simulink model "qbot_platform_alpha_driver_physical"  (R2024a)
settings: Solver=ode1  StartTime=0.0  StopTime=inf  FixedStep=1/480  RelTol=1e-3  EnableMultiTasking=on
undefined symbols (not defined in the file): HIL, qc_get_step_size
libraries: quarc_library x26, simulink x14
settings Model: SimulationMode=external  ExtModeTrigDuration=10000  Creator=mbohra  LastModifiedBy=mbohra
settings SolverCC: AlgebraicLoopSolver=TrustRegion  PositivePriorityOrder=on
settings DataIOCC: ReturnWorkspaceOutputs=off
settings OptimizationCC: ReuseModelBlockBuffer=off
settings DebuggingCC: UnconnectedInputMsg=warning  UnconnectedOutputMsg=warning  UnconnectedLineMsg=warning  ArithmeticOperatorsInVariantConditions=warning
settings HardwareCC: ProdBitPerLong=64  ProdLargestAtomicInteger=LongLong  ProdLargestAtomicFloat=Double  ProdLongLongMode=on  ProdHWDeviceType=ARM Compatible->ARM 64-bit (LP64)
settings ModelReferenceCC: EnableRefExpFcnMdlSchedulingChecks=on
settings SFSimCC: SimUseLocalCustomCode=off  CustomCodeUndefinedFunction=UseInterfaceOnly
settings RTWCC: Description=QUARC Linux Raspberry Pi Arm64 Target (QBot Platform Alpha) Using Toolchain  SystemTargetFile=quarc_linux_pi_arm64.tlc  TemplateMakefile=quarc_default_tmf  RTWUseLocalCustomCode=off  Toolchain=QUARC linux_pi_arm64 | gmake (64-bit Windows)  BuildConfiguration=Faster Runs  GPUComputeCapability=3.5
settings CodeAppCC: StateflowObjectComments=on
settings STFCustomTargetCC: ConcurrentExecutionCompliant=on  SystemTargetFile=quarc_linux_pi_arm64.tlc
settings GRTTargetCC: ParMdlRefBuildCompliant=off  CompOptLevelCompliant=off  CombineOutputUpdateFcns=off  MatFileLogging=off  CPPClassGenCompliant=off  GRTInterface=on  ExtMode=on  ExtModeMexFile=quarc_comm  ExtModeMexArgs='-w -d /tmp -uri %u', 'tcpip://192.168.3.29:17099'
settings ConfigComp: CovMetricSettings=dswe

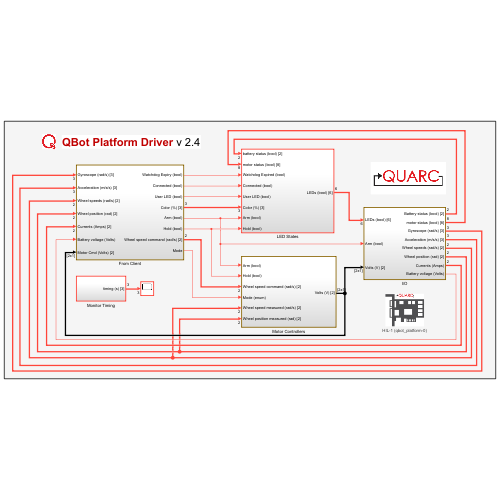
[thumbnail: Simulink's stored preview of the top-level diagram]
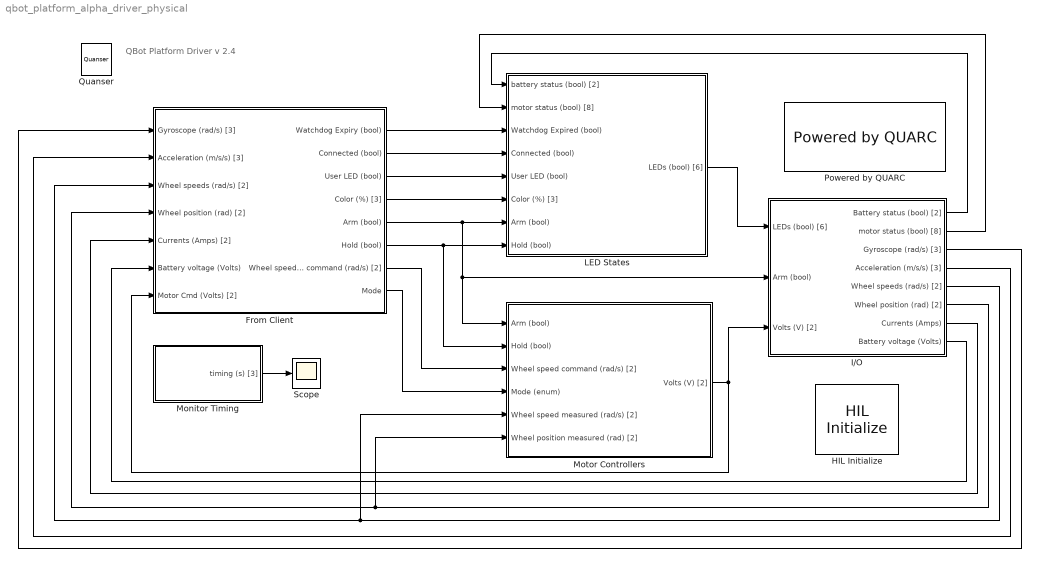
== system qbot_platform_alpha_driver_physical ==
  note: QBot Platform Driver v 2.4
  From Client : Subsystem
  HIL Initialize : quarc_library/Data Acquisition/Generic/Configuration/HIL Initialize  object_name=HIL-1  board_type=qbot_platform  board_number=0  board_options=usb_update_rate=0.002  exclusive=off  active=on  hardware_clocks=[]  clock_modes=[]  initial_clock_frequencies=[]  set_clock_params_at_start=off  set_clock_params_at_switch_in=off  set_clock_frequencies_at_start=off  set_clock_frequencies_at_switch_in=off  analog_input_channels=[0:5]  analog_input_configurations=[]  analog_input_maximums=[18.0 18.0 16.5 16.5 16.5 18.0]  analog_input_minimums=[0 0 0 0 0 0]  set_analog_input_params_at_start=off  set_analog_input_params_at_switch_in=off  analog_output_channels=[]  analog_output_maximums=[]  analog_output_minimums=[]  initial_analog_outputs=[]  final_analog_outputs=[]  watchdog_analog_outputs=[]  set_analog_output_params_at_start=off  set_analog_output_params_at_switch_in=off  set_analog_outputs_at_start=off  set_analog_outputs_at_switch_in=off  set_analog_outputs_at_terminate=off  set_analog_outputs_at_switch_out=off  set_analog_outputs_on_watchdog=off  digital_input_channels=[28:40]  digital_output_channels=[28:30]  digital_output_configuration=[]  initial_digital_outputs=[1]  final_digital_outputs=[0]  watchdog_digital_outputs=[0]  set_digital_output_params_at_start=off  set_digital_output_params_at_switch_in=off  set_digital_outputs_at_start=on  set_digital_outputs_at_switch_in=off  set_digital_outputs_at_terminate=on  set_digital_outputs_at_switch_out=off  set_digital_outputs_on_watchdog=on  encoder_channels=[0:1]  quadrature=[4]  encoder_filter_frequency=[]  initial_encoder_counts=[0]  set_encoder_params_at_start=on  set_encoder_params_at_switch_in=off  set_encoder_counts_at_start=on  set_encoder_counts_at_switch_in=off  pwm_channels=[0:1]  pwm_modes=0  pwm_frequency=[4095 4095]  pwm_configuration=[0]  pwm_alignment=[0]  pwm_polarity=[1]  pwm_leading_deadband=[]  pwm_trailing_deadband=[]  initial_pwm_outputs=[0]  final_pwm_outputs=[0]  watchdog_pwm_outputs=[0]  set_pwm_params_at_start=on  set_pwm_params_at_switch_in=off  set_pwm_outputs_at_start=on  set_pwm_outputs_at_switch_in=off  set_pwm_outputs_at_terminate=on  set_pwm_outputs_at_switch_out=off  set_pwm_outputs_on_watchdog=on  other_output_channels=[11000:11005]  initial_other_outputs=[0 1 0 0 1 0]  final_other_outputs=[1 0 0 1 0 0]  watchdog_other_outputs=[0 0 1 0 0 1]  set_other_outputs_at_start=on  set_other_outputs_at_switch_in=off  set_other_outputs_at_terminate=on  set_other_outputs_at_switch_out=off  set_other_outputs_on_watchdog=on
  I/O : Subsystem
  LED States : Subsystem
  Monitor Timing : Subsystem
  Motor Controllers : Subsystem
  Powered by QUARC : quarc_library/Logos/Powered by QUARC
  Quanser : quarc_library/Logos/Quanser
  Scope : Scope
  wires:
  Monitor Timing/1(timing (s) [3]) -> Scope/1
  From Client/8(Mode) -> Motor Controllers/4(Mode (enum))
  I/O/3(Gyroscope (rad/s) [3]) -> From Client/1(Gyroscope (rad/s) [3])
  I/O/4(Acceleration (m/s/s) [3]) -> From Client/2(Acceleration (m/s/s) [3])
  From Client/5(Arm (bool)) -> Motor Controllers/1(Arm (bool)), I/O/2(Arm (bool)), LED States/7(Arm (bool))
  From Client/3(User LED (bool)) -> LED States/5(User LED (bool))
  From Client/2(Connected (bool)) -> LED States/4(Connected (bool))
  From Client/1(Watchdog Expiry (bool)) -> LED States/3(Watchdog Expired (bool))
  From Client/4(Color (%) [3]) -> LED States/6(Color (%) [3])
  From Client/6(Hold (bool)) -> Motor Controllers/2(Hold (bool)), LED States/8(Hold (bool))
  LED States/1(LEDs (bool) [6]) -> I/O/1(LEDs (bool) [6])
  I/O/5(Wheel speeds (rad/s) [2]) -> Motor Controllers/5(Wheel speed measured (rad/s) [2]), From Client/3(Wheel speeds (rad/s) [2])
  I/O/6(Wheel position (rad) [2]) -> Motor Controllers/6(Wheel position measured (rad) [2]), From Client/4(Wheel position (rad) [2])
  Motor Controllers/1(Volts (V) [2]) -> I/O/3(Volts (V) [2]), From Client/7(Motor Cmd (Volts) [2])
  From Client/7(Wheel speed command (rad/s) [2]) -> Motor Controllers/3(Wheel speed command (rad/s) [2])
  I/O/1(Battery status (bool) [2]) -> LED States/1(battery status (bool) [2])
  I/O/2(motor status (bool) [8]) -> LED States/2(motor status (bool) [8])
  I/O/7(Currents (Amps)) -> From Client/5(Currents (Amps) [2])
  I/O/8(Battery voltage (Volts)) -> From Client/6(Battery voltage (Volts))

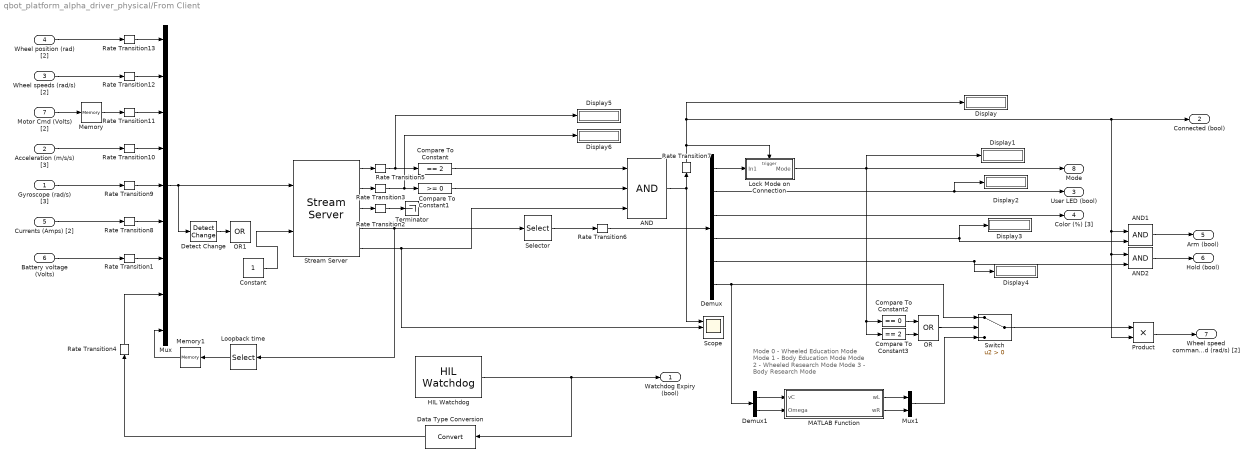
== system qbot_platform_alpha_driver_physical/From Client ==
  note: Mode 0 - Wheeled Education Mode
      | Mode 1 - Body Education Mode
      | Mode 2 - Wheeled Research Mode
      | Mode 3 - Body Research Mode
  Gyroscope (rad/s) [3] : Inport
  Acceleration (m/s/s) [3] : Inport  Port=2
  Wheel speeds (rad/s) [2] : Inport  Port=3
  Wheel position (rad) [2] : Inport  Port=4
  Currents (Amps) [2] : Inport  Port=5
  Battery voltage (Volts) : Inport  Port=6
  Motor Cmd (Volts) [2] : Inport  Port=7
  AND : Logic  Inputs=3  IconShape=distinctive  AllPortsSameDT=off  OutDataTypeStr=boolean
  AND1 : Logic  IconShape=distinctive  AllPortsSameDT=off  OutDataTypeStr=boolean
  AND2 : Logic  IconShape=distinctive  AllPortsSameDT=off  OutDataTypeStr=boolean
  Compare To Constant : simulink/Logic and Bit Operations/Compare To Constant  relop===  const=2  OutDataTypeStr=boolean
  Compare To Constant1 : simulink/Logic and Bit Operations/Compare To Constant  relop=>=  const=0  OutDataTypeStr=boolean
  Compare To Constant2 : simulink/Logic and Bit Operations/Compare To Constant  relop===  const=0  OutDataTypeStr=boolean
  Compare To Constant3 : simulink/Logic and Bit Operations/Compare To Constant  relop===  const=2  OutDataTypeStr=boolean
  Constant : Constant
  Data Type Conversion : DataTypeConversion  SaturateOnIntegerOverflow=off  RndMeth=Floor
  Demux : Demux  Outputs=[1 1 3 1 1 2]
  Demux1 : Demux  Outputs=2
  Detect Change : simulink/Logic and Bit Operations/Detect Change  vinit=0  OutDataTypeStr=boolean
  Display{,1..6} (7 alike) : Display
  HIL Watchdog : quarc_library/Data Acquisition/Generic/Watchdog/HIL Watchdog  object_name=HIL-1  timeout=0.1  sample_time=qc_get_step_size  active=off
      settings: AttributesFormatString=(%<object_name>)  SourceProductName=QUARC Targets
  Lock Mode on Connection : Subsystem  TreatAsAtomicUnit=on
  Loopback time : Selector  InputPortWidth=10  IndexOptions=Index vector (dialog)  Indices=10  OutputSizes=1
  MATLAB Function : MATLAB Function  TreatAsAtomicUnit=on
  Memory : Memory
  Memory1 : Memory  InheritSampleTime=on
  Mux : Mux  Inputs=9
  Mux1 : Mux  Inputs=2
  OR : Logic  Operator=OR  IconShape=distinctive  AllPortsSameDT=off  OutDataTypeStr=boolean
  OR1 : Logic  Operator=OR  Inputs=1  IconShape=distinctive  AllPortsSameDT=off
  Product : Product
  Rate Transition{1..13} (13 alike) : RateTransition
  Scope : Scope  NumInputPorts=3
  Selector : Selector  InputPortWidth=10  IndexOptions=Index vector (dialog)  Indices=1:9  OutputSizes=1
  Stream Server : quarc_library/Communications/Basic/Stream Server  uri_source=Specify via dialog (do not evaluate)  uri=tcpip://localhost:18888?nagle='off'  send_buffer_size=1460  receive_buffer_size=1460  byte_order=little endian (Intel - LSB first)  optimization=Minimum latency  send_options=Send most recent data  receive_options=Receive most recent data  default_value=zeros(10,1)  sample_time=qc_get_step_size*8  active=off  implementation=Use blocking I/O in a separate thread  send_fifo_size=1000  receive_fifo_size=1000  send_priority=0  receive_priority=0  send_dimensions=off  receive_dimensions=off  max_dimensions=-1  data_type=Inherited via back propagation  type_expr=BusObject
      settings: AttributesFormatString="\"tcpip://localhost:18888?nagle='off'\""
  Switch : Switch  Criteria=u2 > Threshold  SaturateOnIntegerOverflow=off  InputSameDT=off
  Terminator : Terminator
  Watchdog Expiry (bool) : Outport
  Connected (bool) : Outport  Port=2
  User LED (bool) : Outport  Port=3
  Color (%) [3] : Outport  Port=4
  Arm (bool) : Outport  Port=5
  Hold (bool) : Outport  Port=6
  Wheel speed command (rad/s) [2] : Outport  Port=7
  Mode : Outport  Port=8
  wires:
  HIL Watchdog/1 -> Data Type Conversion/1, Watchdog Expiry (bool)/1
  Demux/3 -> Color (%) [3]/1
  Demux/5 -> AND2/2, Display4/1
  Demux/2 -> Display2/1, User LED (bool)/1
  Demux/6 -> Demux1/1, Switch/1
  Stream Server/2 -> Rate Transition3/1
  Stream Server/1 -> Rate Transition5/1
  Compare To Constant1/1 -> AND/2
  Compare To Constant/1 -> AND/1
  Gyroscope (rad/s) [3]/1 -> Rate Transition9/1
  Acceleration (m/s/s) [3]/1 -> Rate Transition10/1
  Wheel position (rad) [2]/1 -> Rate Transition13/1
  Motor Cmd (Volts) [2]/1 -> Memory/1
  Detect Change/1 -> OR1/1
  Stream Server/3 -> Rate Transition2/1
  Lock Mode on Connection/1(Mode) -> Mode/1, Display1/1, Compare To Constant3/1, Compare To Constant2/1
  Data Type Conversion/1 -> Rate Transition4/1
  Memory/1 -> Rate Transition11/1
  Compare To Constant2/1 -> OR/1
  Compare To Constant3/1 -> OR/2
  OR/1 -> Switch/2
  Mux1/1 -> Switch/3
  Demux/1 -> Lock Mode on Connection/1(In1)
  MATLAB Function/1(wL) -> Mux1/1
  MATLAB Function/2(wR) -> Mux1/2
  Selector/1 -> Rate Transition6/1
  Loopback time/1 -> Memory1/1
  Memory1/1 -> Mux/9
  Switch/1 -> Product/1
  Wheel speeds (rad/s) [2]/1 -> Rate Transition12/1
  Demux/4 -> AND1/2, Display3/1
  AND/1 -> Scope/1, Rate Transition7/1
  Demux1/1 -> MATLAB Function/1(vC)
  Demux1/2 -> MATLAB Function/2(Omega)
  AND2/1 -> Hold (bool)/1
  Currents (Amps) [2]/1 -> Rate Transition8/1
  Battery voltage (Volts)/1 -> Rate Transition1/1
  Product/1 -> Wheel speed command (rad/s) [2]/1
  AND1/1 -> Arm (bool)/1
  Stream Server/5 -> AND/3, Scope/2
  Stream Server/4 -> Selector/1, Loopback time/1
  Rate Transition2/1 -> Terminator/1
  Rate Transition3/1 -> Display6/1, Compare To Constant1/1
  Rate Transition5/1 -> Display5/1, Compare To Constant/1
  Constant/1 -> Stream Server/2
  Mux/1 -> Stream Server/1, Detect Change/1
  Rate Transition1/1 -> Mux/7
  Rate Transition8/1 -> Mux/6
  Rate Transition9/1 -> Mux/5
  Rate Transition10/1 -> Mux/4
  Rate Transition11/1 -> Mux/3
  Rate Transition12/1 -> Mux/2
  Rate Transition13/1 -> Mux/1
  Rate Transition6/1 -> Demux/1
  Rate Transition7/1 -> Lock Mode on Connection/Trigger, Product/2, AND2/1, AND1/1, Connected (bool)/1, Display/1
  Rate Transition4/1 -> Mux/8

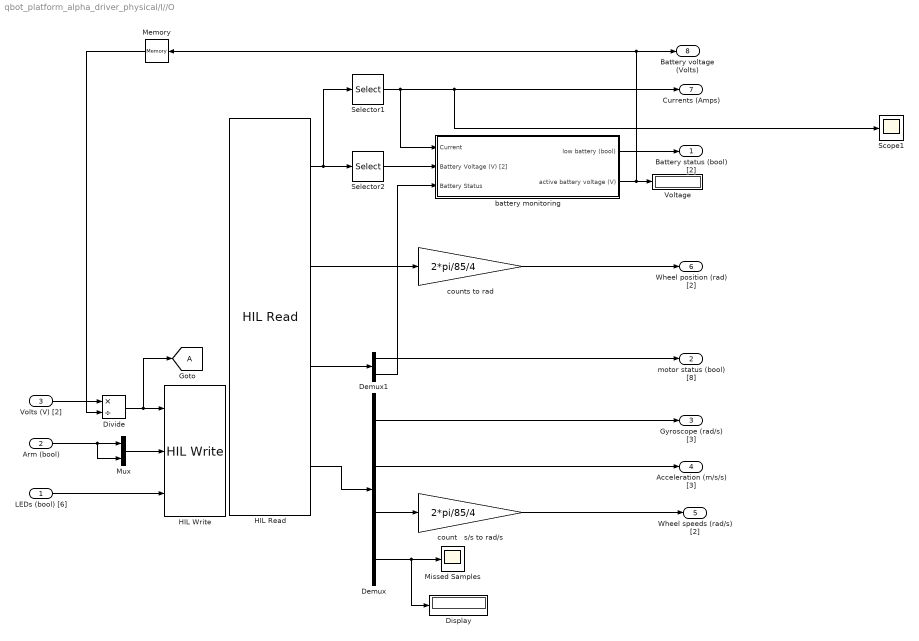
== system qbot_platform_alpha_driver_physical/I//O ==
  LEDs (bool) [6] : Inport
  Arm (bool) : Inport  Port=2
  Volts (V) [2] : Inport  Port=3
  Demux : Demux  Outputs=[3 3 2 1]
  Demux1 : Demux  Outputs=[8 2]
  Display : Display
  Divide : Product  Inputs=*/
  Goto : Goto  TagVisibility=global
  HIL Read : quarc_library/Data Acquisition/Generic/Immediate I//O/HIL Read  object_name=HIL-1  analog_channels=[0:3]  encoder_channels=[0:1]  digital_channels=[28:29 32:33 30:31 34:35 39:40]  other_channels=[3000:3002 4000:4002 14000:14001 13000]  sample_time=qc_get_step_size  active=on  vector_output=on  data_type_mode=Inherit via back propagation  encoder_data_type=double  digital_data_type=boolean
  HIL Write : quarc_library/Data Acquisition/Generic/Immediate I//O/HIL Write  object_name=HIL-1  analog_channels=[]  pwm_channels=[0:1]  digital_channels=[28:29]  other_channels=[11000:11005]  sample_time=-1  active=off  vector_input=on
  Memory : Memory  InitialCondition=13.5
  Missed Samples : Scope
  Mux : Mux  Inputs=2
  Scope1 : Scope
  Selector1 : Selector  InputPortWidth=4  IndexOptions=Index vector (dialog)  Indices=3:4  OutputSizes=1
  Selector2 : Selector  InputPortWidth=4  IndexOptions=Index vector (dialog)  Indices=1:2  OutputSizes=1
  Voltage : Display
  battery monitoring : Subsystem
  count   s/s to rad/s : Gain  Gain=2*pi/85/4
  counts to rad : Gain  Gain=2*pi/85/4
  Battery status (bool) [2] : Outport
  motor status (bool) [8] : Outport  Port=2
  Gyroscope (rad/s) [3] : Outport  Port=3
  Acceleration (m/s/s) [3] : Outport  Port=4
  Wheel speeds (rad/s) [2] : Outport  Port=5
  Wheel position (rad) [2] : Outport  Port=6
  Currents (Amps) : Outport  Port=7
  Battery voltage (Volts) : Outport  Port=8
  wires:
  HIL Read/2 -> counts to rad/1
  HIL Read/4 -> Demux/1
  Volts (V) [2]/1 -> Divide/1
  LEDs (bool) [6]/1 -> HIL Write/3
  counts to rad/1 -> Wheel position (rad) [2]/1
  Demux/3 -> count   s/s to rad/s/1
  Demux/1 -> Gyroscope (rad/s) [3]/1
  Demux/2 -> Acceleration (m/s/s) [3]/1
  count   s/s to rad/s/1 -> Wheel speeds (rad/s) [2]/1
  HIL Read/1 -> Selector1/1, Selector2/1
  battery monitoring/1(low battery (bool)) -> Battery status (bool) [2]/1
  HIL Read/3 -> Demux1/1
  Selector2/1 -> battery monitoring/2(Battery Voltage (V) [2])
  Selector1/1 -> battery monitoring/1(Current), Scope1/1, Currents (Amps)/1
  Demux/4 -> Display/1, Missed Samples/1
  battery monitoring/2(active battery voltage (V)) -> Memory/1, Battery voltage (Volts)/1, Voltage/1
  Arm (bool)/1 -> Mux/2, Mux/1
  Mux/1 -> HIL Write/2
  Memory/1 -> Divide/2
  Divide/1 -> Goto/1, HIL Write/1
  Demux1/2 -> battery monitoring/3(Battery Status)
  Demux1/1 -> motor status (bool) [8]/1

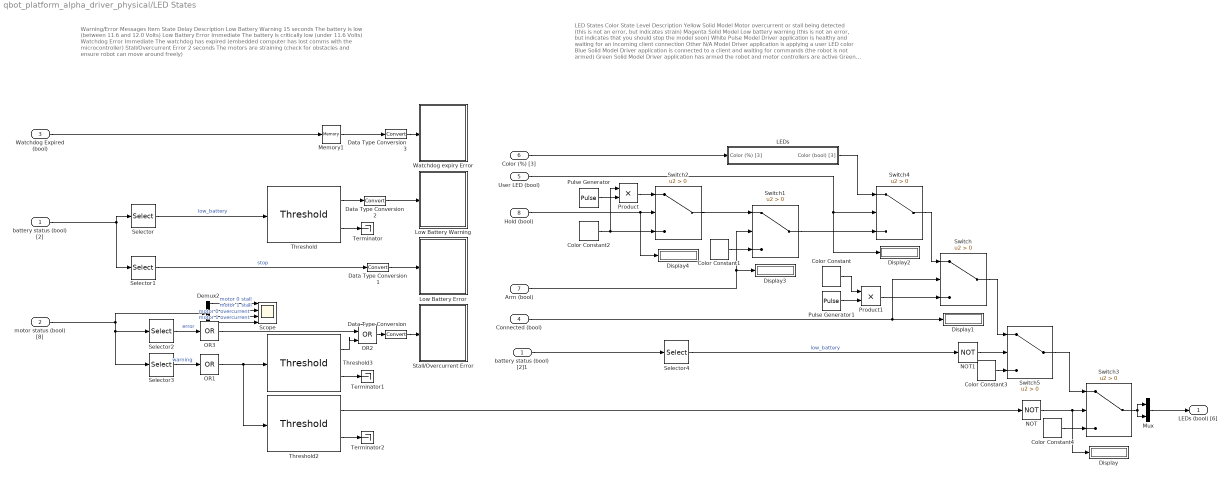
== system qbot_platform_alpha_driver_physical/LED States ==
  note: LED States
      |
      | Color State Level Description
      | Yellow Solid Model Motor overcurrent or stall being detected (this is not an error, but indicates strain)
      | Magenta Solid Model Low battery warning (this is not an error, but indicates that you should stop the model soon)
      | White Pulse Model Driver application is healthy and waiting for an incoming client connection
      | Other N/A Model Driver application is applying a user LED color
      | Blue Solid Model Driver application is connected to a client and waiting for commands (the robot is not armed)
      | Green Solid Model Driver application has armed the robot and motor controllers are active
      | Green Pulse Model Driver application has armed the robot and is attempting to hold the robot's position
      | Red Solid Firmware Driver application was stopped normally without any error conditions
      | Red Pulse Firmware Embedded Computer has shutdown and the robot must be turned OFF using the power switch.
  note: Warning/Error Messages
      |
      | Item State Delay Description
      | Low Battery Warning 15 seconds The battery is low (between 11.6 and 12.0 Volts)
      | Low Battery Error Immediate The battery is critically low (under 11.6 Volts)
      | Watchdog Error Immediate The watchdog has expired (embedded computer has lost comms with the microcontroller)
      | Stall/Overcurrent Error 2 seconds The motors are straining (check for obstacles and ensure robot can move around freely)
  battery status (bool) [2] : Inport
  motor status (bool) [8] : Inport  Port=2
  Watchdog Expired (bool) : Inport  Port=3
  Connected (bool) : Inport  Port=4
  User LED (bool) : Inport  Port=5
  Color (%) [3] : Inport  Port=6
  Arm (bool) : Inport  Port=7
  Hold (bool) : Inport  Port=8
  Color Constant : quarc_library/Sources/Signals/Color Constant  color=[1 1 1]
      settings: SourceProductName=QUARC Targets
  Color Constant1 : quarc_library/Sources/Signals/Color Constant  color=[0 0 1]
      settings: SourceProductName=QUARC Targets
  Color Constant2 : quarc_library/Sources/Signals/Color Constant  color=[0 1 0]
      settings: SourceProductName=QUARC Targets
  Color Constant3 : quarc_library/Sources/Signals/Color Constant  color=[1 0 1]
      settings: SourceProductName=QUARC Targets
  Color Constant4 : quarc_library/Sources/Signals/Color Constant  color=[1 1 0]
      settings: SourceProductName=QUARC Targets
  Data Type Conversion{,1..3} (4 alike) : DataTypeConversion  SaturateOnIntegerOverflow=off  RndMeth=Floor
  Demux2 : Demux  Outputs=[2 2 2 2]
  Display{,1..4} (5 alike) : Display
  LEDs : Subsystem
  Low Battery Error : Subsystem
  Low Battery Warning : Subsystem
  Memory1 : Memory
  Mux : Mux  Inputs=2
  NOT : Logic  Operator=NOT  IconShape=distinctive  AllPortsSameDT=off  OutDataTypeStr=boolean
  NOT1 : Logic  Operator=NOT  IconShape=distinctive  AllPortsSameDT=off  OutDataTypeStr=boolean
  OR1 : Logic  Operator=OR  Inputs=1  IconShape=distinctive  AllPortsSameDT=off  OutDataTypeStr=boolean
  OR2 : Logic  Operator=OR  IconShape=distinctive  AllPortsSameDT=off  OutDataTypeStr=boolean
  OR3 : Logic  Operator=OR  Inputs=1  IconShape=distinctive  AllPortsSameDT=off  OutDataTypeStr=boolean
  Product : Product
  Product1 : Product
  Pulse Generator : DiscretePulseGenerator  PulseType=Time based  Period=1  PulseWidth=70
  Pulse Generator1 : DiscretePulseGenerator  PulseType=Time based  Period=1  PulseWidth=30
  Scope : Scope  NumInputPorts=4
  Selector : Selector  InputPortWidth=2  IndexOptions=Index vector (dialog)  Indices=1  OutputSizes=1
  Selector1 : Selector  InputPortWidth=2  IndexOptions=Index vector (dialog)  Indices=2  OutputSizes=1
  Selector2 : Selector  InputPortWidth=8  IndexOptions=Index vector (dialog)  Indices=[2 4 6 8]  OutputSizes=1
  Selector3 : Selector  InputPortWidth=8  IndexOptions=Index vector (dialog)  Indices=[1 3 5 7]  OutputSizes=1
  Selector4 : Selector  InputPortWidth=2  IndexOptions=Index vector (dialog)  Indices=1  OutputSizes=1
  Stall/Overcurrent Error : Subsystem
  Switch{,1..5} (6 alike) : Switch  Criteria=u2 > Threshold  SaturateOnIntegerOverflow=off  InputSameDT=off
  Terminator : Terminator
  Terminator1 : Terminator
  Terminator2 : Terminator
  Threshold : quarc_library/Discontinuities/Threshold  operator=>=  param_src=Specify via dialog  threshold=0.5  duration=15
      settings: SourceProductName=QUARC Targets
  Threshold2 : quarc_library/Discontinuities/Threshold  operator=>=  param_src=Specify via dialog  threshold=0.5  duration=0.75
      settings: SourceProductName=QUARC Targets
  Threshold3 : quarc_library/Discontinuities/Threshold  operator=>=  param_src=Specify via dialog  threshold=0.5  duration=2
      settings: SourceProductName=QUARC Targets
  Watchdog expiry Error : Subsystem
  battery status (bool) [2]1 : InportShadow
  LEDs (bool) [6] : Outport
  wires:
  Connected (bool)/1 -> Display1/1, Switch/2
  Product1/1 -> Switch/3
  Arm (bool)/1 -> Switch1/2, Display3/1
  Mux/1 -> LEDs (bool) [6]/1
  Color Constant1/1 -> Switch1/3
  Switch2/1 -> Switch1/1
  Hold (bool)/1 -> Display4/1, Switch2/2
  Color Constant2/1 -> Product/1, Switch2/3
  Product/1 -> Switch2/1
  Watchdog Expired (bool)/1 -> Memory1/1
  Color Constant4/1 -> Switch3/3
  NOT/1 -> Display/1, Switch3/2
  Pulse Generator/1 -> Product/2
  Switch4/1 -> Switch/1
  Switch1/1 -> Switch4/3
  User LED (bool)/1 -> Switch4/2, Display2/1
  Color (%) [3]/1 -> LEDs/1(Color (%) [3])
  LEDs/1(Color (bool) [3]) -> Switch4/1
  Switch/1 -> Switch5/1
  battery status (bool) [2]/1 -> Selector/1, Selector1/1
  NOT1/1 -> Switch5/2
  Color Constant3/1 -> Switch5/3
  Switch3/1 -> Mux/2, Mux/1
  Switch5/1 -> Switch3/1
  motor status (bool) [8]/1 -> Demux2/1, Selector3/1, Selector2/1
  Threshold/1 -> Data Type Conversion2/1
  Memory1/1 -> Data Type Conversion3/1
  Threshold/2 -> Terminator/1
  Selector/1 -> Threshold/1  "low_battery"
  Selector1/1 -> Data Type Conversion1/1  "stop"
  Demux2/1 -> Scope/1  "motor 0 stall"
  Demux2/4 -> Scope/4  "motor 1 overcurrent"
  Demux2/2 -> Scope/2  "motor 1 stall"
  Demux2/3 -> Scope/3  "motor 0 overcurrent"
  Selector3/1 -> OR1/1  "warning"
  Selector2/1 -> OR3/1  "error"
  OR1/1 -> Threshold3/1, Threshold2/1
  Threshold3/1 -> OR2/2
  OR2/1 -> Data Type Conversion/1
  Threshold3/2 -> Terminator1/1
  Threshold2/2 -> Terminator2/1
  Pulse Generator1/1 -> Product1/2
  Color Constant/1 -> Product1/1
  battery status (bool) [2]1/1 -> Selector4/1
  Selector4/1 -> NOT1/1  "low_battery"
  Threshold2/1 -> NOT/1
  OR3/1 -> OR2/1
  Data Type Conversion/1 -> Stall/Overcurrent Error/Trigger
  Data Type Conversion1/1 -> Low Battery Error/Trigger
  Data Type Conversion2/1 -> Low Battery Warning/Trigger
  Data Type Conversion3/1 -> Watchdog expiry Error/Trigger

== system qbot_platform_alpha_driver_physical/Monitor Timing ==
  Computation Time : quarc_library/Sources/Time/Computation Time  sample_time=qc_get_step_size  use_model=on  use_cpu_time=off
  Constant : Constant  Value=qc_get_step_size
  Mux : Mux  Inputs=3
  Sample Time : quarc_library/Sources/Time/Sample Time  Priority=-99  sample_time=qc_get_step_size
  timing (s) [3] : Outport
  wires:
  Sample Time/1 -> Mux/1  "achieved sample time"
  Computation Time/1 -> Mux/3  "computation time"
  Mux/1 -> timing (s) [3]/1
  Constant/1 -> Mux/2  "target sample time"

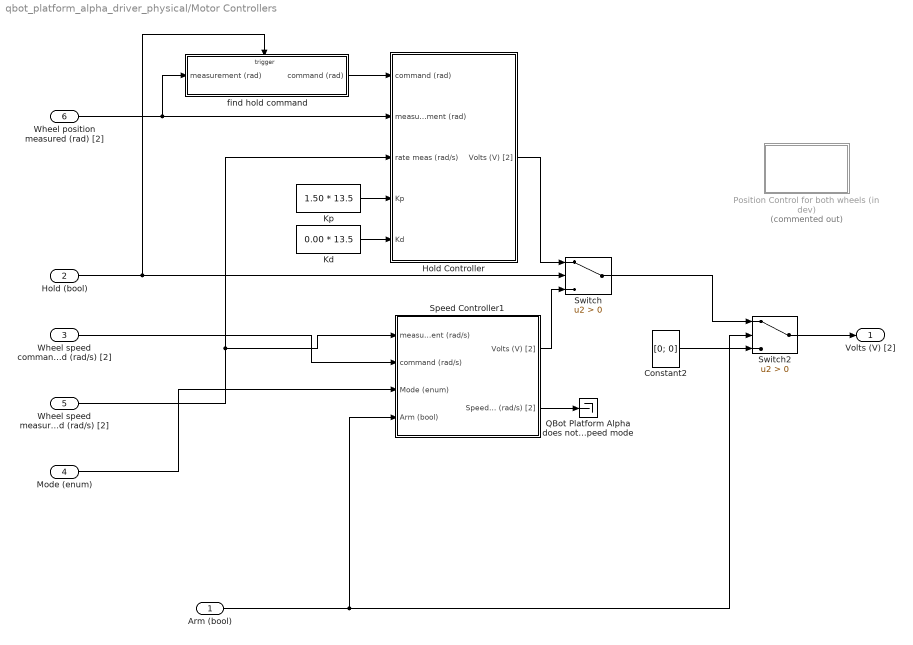
== system qbot_platform_alpha_driver_physical/Motor Controllers ==
  Arm (bool) : Inport
  Hold (bool) : Inport  Port=2
  Wheel speed command (rad/s) [2] : Inport  Port=3
  Mode (enum) : Inport  Port=4
  Wheel speed measured (rad/s) [2] : Inport  Port=5
  Wheel position measured (rad) [2] : Inport  Port=6
  Constant2 : Constant  Value=[0; 0]  VectorParams1D=off
  Hold Controller : Subsystem
  "Kd " : Constant  Value=0.00 * 13.5
  "Kp " : Constant  Value=1.50 * 13.5
  Position Control for both wheels (in dev) : Subsystem  Commented=on
  QBot Platform Alpha does not support Speed mode : Terminator
  Speed Controller1 : Subsystem
  Switch : Switch  Criteria=u2 > Threshold  SaturateOnIntegerOverflow=off  InputSameDT=off
  Switch2 : Switch  Criteria=u2 > Threshold  SaturateOnIntegerOverflow=off  InputSameDT=off
  find hold command : Subsystem  TreatAsAtomicUnit=on
  Volts (V) [2] : Outport
  wires:
  Constant2/1 -> Switch2/3
  Hold (bool)/1 -> Switch/2, find hold command/Trigger
  Switch/1 -> Switch2/1
  Speed Controller1/1(Volts (V) [2]) -> Switch/3
  Arm (bool)/1 -> Speed Controller1/4(Arm (bool)), Switch2/2
  "Kp "/1 -> Hold Controller/4(Kp)
  Wheel speed command (rad/s) [2]/1 -> Speed Controller1/2(command (rad/s))
  find hold command/1(command (rad)) -> Hold Controller/1(command (rad))
  Wheel position measured (rad) [2]/1 -> find hold command/1(measurement (rad)), Hold Controller/2(measurement (rad))
  Wheel speed measured (rad/s) [2]/1 -> Speed Controller1/1(measurement (rad/s)), Hold Controller/3(rate meas (rad/s))
  Switch2/1 -> Volts (V) [2]/1
  Mode (enum)/1 -> Speed Controller1/3(Mode (enum))
  Hold Controller/1(Volts (V) [2]) -> Switch/1
  "Kd "/1 -> Hold Controller/5(Kd)
  Speed Controller1/2(Speed Cmd (rad/s) [2]) -> QBot Platform Alpha does not support Speed mode/1

== system qbot_platform_alpha_driver_physical/From Client/Lock Mode on Connection ==
  In1 : Inport
  Trigger : TriggerPort  VariantControl=(inherit)
  Mode : Outport
  wires:
  In1/1 -> Mode/1

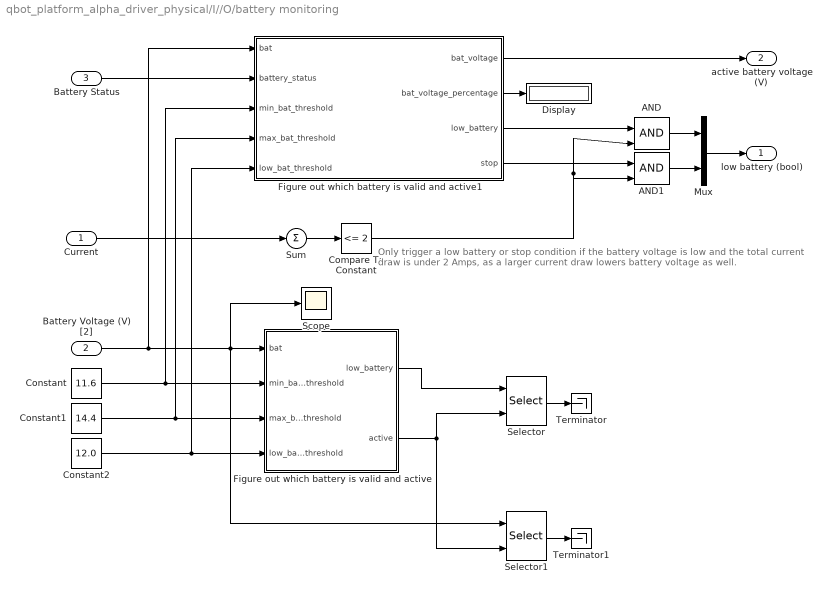
== system qbot_platform_alpha_driver_physical/I//O/battery monitoring ==
  note: Only trigger a low battery or stop condition if the battery voltage is low and the total current draw is under 2 Amps, as a larger current draw lowers battery voltage as well.
  Current : Inport
  Battery Voltage (V) [2] : Inport  Port=2
  Battery Status : Inport  Port=3
  AND : Logic  IconShape=distinctive  AllPortsSameDT=off  OutDataTypeStr=boolean
  AND1 : Logic  IconShape=distinctive  AllPortsSameDT=off  OutDataTypeStr=boolean
  Compare To Constant : simulink/Logic and Bit Operations/Compare To Constant  relop=<=  const=2  OutDataTypeStr=boolean
  Constant : Constant  Value=11.6
  Constant1 : Constant  Value=14.4
  Constant2 : Constant  Value=12.0
  Display : Display
  Figure out which battery is valid and active : MATLAB Function  TreatAsAtomicUnit=on
  Figure out which battery is valid and active1 : MATLAB Function  TreatAsAtomicUnit=on
  Mux : Mux  Inputs=2
  Scope : Scope
  Selector : Selector  InputPortWidth=2  IndexOptions=Index vector (port)  Indices=[1 3]  OutputSizes=1
  Selector1 : Selector  InputPortWidth=2  IndexOptions=Index vector (port)  Indices=[1 3]  OutputSizes=1
  Sum : Sum  Inputs=1
  Terminator : Terminator
  Terminator1 : Terminator
  low battery (bool) : Outport
  active battery voltage (V) : Outport  Port=2
  wires:
  Battery Voltage (V) [2]/1 -> Figure out which battery is valid and active1/1(bat), Scope/1, Selector1/1, Figure out which battery is valid and active/1(bat)
  Figure out which battery is valid and active/1(low_battery) -> Selector/1
  Figure out which battery is valid and active/2(active) -> Selector/2, Selector1/2
  Constant/1 -> Figure out which battery is valid and active1/3(min_bat_threshold), Figure out which battery is valid and active/2(min_bat_threshold)
  Constant1/1 -> Figure out which battery is valid and active1/4(max_bat_threshold), Figure out which battery is valid and active/3(max_bat_threshold)
  Constant2/1 -> Figure out which battery is valid and active1/5(low_bat_threshold), Figure out which battery is valid and active/4(low_bat_threshold)
  Current/1 -> Sum/1
  Sum/1 -> Compare To Constant/1
  Compare To Constant/1 -> AND1/2, AND/2
  Battery Status/1 -> Figure out which battery is valid and active1/2(battery_status)
  Figure out which battery is valid and active1/3(low_battery) -> AND/1
  Figure out which battery is valid and active1/1(bat_voltage) -> active battery voltage (V)/1
  Figure out which battery is valid and active1/2(bat_voltage_percentage) -> Display/1
  Figure out which battery is valid and active1/4(stop) -> AND1/1
  Mux/1 -> low battery (bool)/1
  AND/1 -> Mux/1
  AND1/1 -> Mux/2
  Selector/1 -> Terminator/1
  Selector1/1 -> Terminator1/1

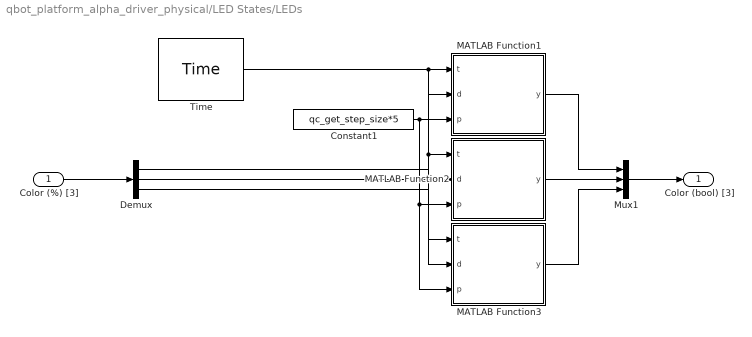
== system qbot_platform_alpha_driver_physical/LED States/LEDs ==
  Color (%) [3] : Inport
  Constant1 : Constant  Value=qc_get_step_size*5
  Demux : Demux  Outputs=3
  MATLAB Function1 : MATLAB Function  TreatAsAtomicUnit=on
  MATLAB Function2 : MATLAB Function  TreatAsAtomicUnit=on
  MATLAB Function3 : MATLAB Function  TreatAsAtomicUnit=on
  Mux1 : Mux  Inputs=3
  Time : quarc_library/Sources/Time/Time  time_source=Wall clock  sample_time=qc_get_step_size
  Color (bool) [3] : Outport
  wires:
  Demux/3 -> MATLAB Function3/2(d)
  Time/1 -> MATLAB Function3/1(t), MATLAB Function2/1(t), MATLAB Function1/1(t)
  MATLAB Function1/1(y) -> Mux1/1
  Constant1/1 -> MATLAB Function3/3(p), MATLAB Function2/3(p), MATLAB Function1/3(p)
  Color (%) [3]/1 -> Demux/1
  Mux1/1 -> Color (bool) [3]/1
  Demux/2 -> MATLAB Function2/2(d)
  MATLAB Function3/1(y) -> Mux1/3
  Demux/1 -> MATLAB Function1/2(d)
  MATLAB Function2/1(y) -> Mux1/2

== system qbot_platform_alpha_driver_physical/LED States/Low Battery Error ==
  Trigger : TriggerPort  VariantControl=(inherit)  ShowOutputPort=on  OutputDataType=double  PortDimensions=1
  Print1 : quarc_library/User Interface/Standard I//O/Print  format_string=ERROR - Low Battery  max_code_units=512  optimization=Minimizing latency  sample_time=-1  active=off
      settings: SourceProductName=QUARC Targets
  Stop with Message3 : quarc_library/Sinks/Error Handling/Stop with Message  message_type=Fixed error message  message_icon=Error  message=ERROR - Low Battery
  Terminator : Terminator
  Terminator1 : Terminator
  wires:
  Print1/1 -> Terminator/1
  Print1/2 -> Terminator1/1
  Trigger/1 -> Stop with Message3/1

== system qbot_platform_alpha_driver_physical/LED States/Low Battery Warning ==
  Trigger : TriggerPort  VariantControl=(inherit)  ShowOutputPort=on  OutputDataType=double  PortDimensions=1
  Print1 : quarc_library/User Interface/Standard I//O/Print  format_string=WARNING - Low Battery  max_code_units=512  optimization=Minimizing latency  sample_time=-1  active=off
      settings: SourceProductName=QUARC Targets
  Stop with Message1 : quarc_library/Sinks/Error Handling/Stop with Message  message_type=Fixed error message  message_icon=Warning  message=WARNING - Low Battery
  Terminator : Terminator
  Terminator1 : Terminator
  wires:
  Print1/1 -> Terminator/1
  Print1/2 -> Terminator1/1
  Trigger/1 -> Stop with Message1/1

== system qbot_platform_alpha_driver_physical/LED States/Stall//Overcurrent Error ==
  Trigger : TriggerPort  VariantControl=(inherit)  ShowOutputPort=on  OutputDataType=double  PortDimensions=1
  Print1 : quarc_library/User Interface/Standard I//O/Print  format_string=ERROR - Stall / Overcurrent  max_code_units=512  optimization=Minimizing latency  sample_time=-1  active=off
      settings: SourceProductName=QUARC Targets
  Stop with Message3 : quarc_library/Sinks/Error Handling/Stop with Message  message_type=Fixed error message  message_icon=Error  message=ERROR - Stall / Overcurrent
  Terminator : Terminator
  Terminator1 : Terminator
  wires:
  Trigger/1 -> Stop with Message3/1
  Print1/2 -> Terminator1/1
  Print1/1 -> Terminator/1

== system qbot_platform_alpha_driver_physical/LED States/Watchdog expiry Error ==
  Trigger : TriggerPort  VariantControl=(inherit)  ShowOutputPort=on  OutputDataType=double  PortDimensions=1
  Print1 : quarc_library/User Interface/Standard I//O/Print  format_string=ERROR - Watchdog expired  max_code_units=512  optimization=Minimizing latency  sample_time=-1  active=off
      settings: SourceProductName=QUARC Targets
  Stop with Message1 : quarc_library/Sinks/Error Handling/Stop with Message  message_type=Fixed error message  message_icon=Warning  message=ERROR - Watchdog expired
  Terminator : Terminator
  Terminator1 : Terminator
  wires:
  Trigger/1 -> Stop with Message1/1
  Print1/2 -> Terminator1/1
  Print1/1 -> Terminator/1

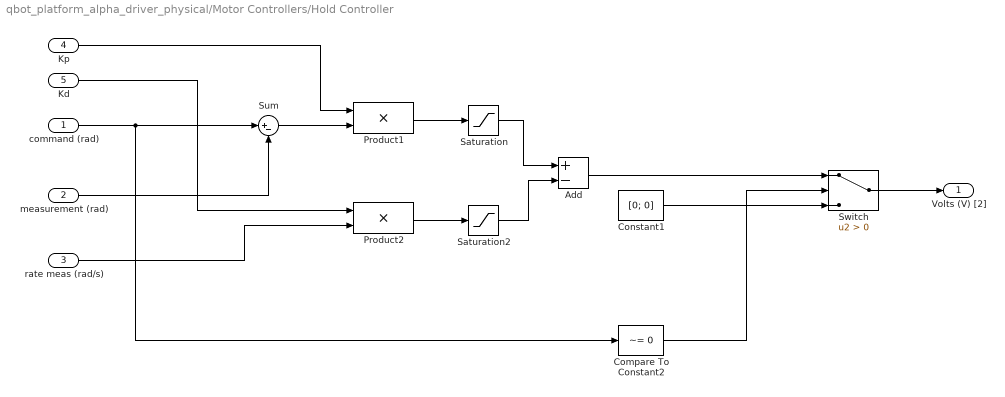
== system qbot_platform_alpha_driver_physical/Motor Controllers/Hold Controller ==
  command (rad) : Inport
  measurement (rad) : Inport  Port=2
  rate meas (rad/s) : Inport  Port=3
  Kp : Inport  Port=4
  Kd : Inport  Port=5
  Add : Sum  Inputs=+-
  Compare To Constant2 : simulink/Logic and Bit Operations/Compare To Constant  relop=~=  const=0  OutDataTypeStr=boolean
  Constant1 : Constant  Value=[0; 0]  VectorParams1D=off
  Product1 : Product
  Product2 : Product
  Saturation : Saturate  UpperLimit=[9.45 9.45]  LowerLimit=[-9.45 -9.45]
  Saturation2 : Saturate  UpperLimit=[4.05 4.05]  LowerLimit=[-4.05 -4.05]
  Sum : Sum  Inputs=|+-
  Switch : Switch  Criteria=u2 > Threshold  SaturateOnIntegerOverflow=off  InputSameDT=off
  Volts (V) [2] : Outport
  wires:
  command (rad)/1 -> Compare To Constant2/1, Sum/1
  measurement (rad)/1 -> Sum/2
  Sum/1 -> Product1/2
  Add/1 -> Switch/1
  Product1/1 -> Saturation/1
  Switch/1 -> Volts (V) [2]/1
  Constant1/1 -> Switch/3
  Kp/1 -> Product1/1
  Compare To Constant2/1 -> Switch/2
  Saturation2/1 -> Add/2
  Saturation/1 -> Add/1
  Product2/1 -> Saturation2/1
  rate meas (rad/s)/1 -> Product2/2
  Kd/1 -> Product2/1

== system qbot_platform_alpha_driver_physical/Motor Controllers/Position Control for both wheels (in dev) ==
  Drive Controller : Subsystem
  "Kd  " : Constant  Value=0.06
  "Ki  " : Constant  Value=0
  "Kp   " : Constant  Value=0.65
  find hold command1 : Subsystem  TreatAsAtomicUnit=on
  wires:
  "Kd  "/1 -> Drive Controller/7(Kd)
  "Ki  "/1 -> Drive Controller/6(Ki)
  find hold command1/1(command (rad)) -> Drive Controller/1(command (rad))
  "Kp   "/1 -> Drive Controller/5(Kp)

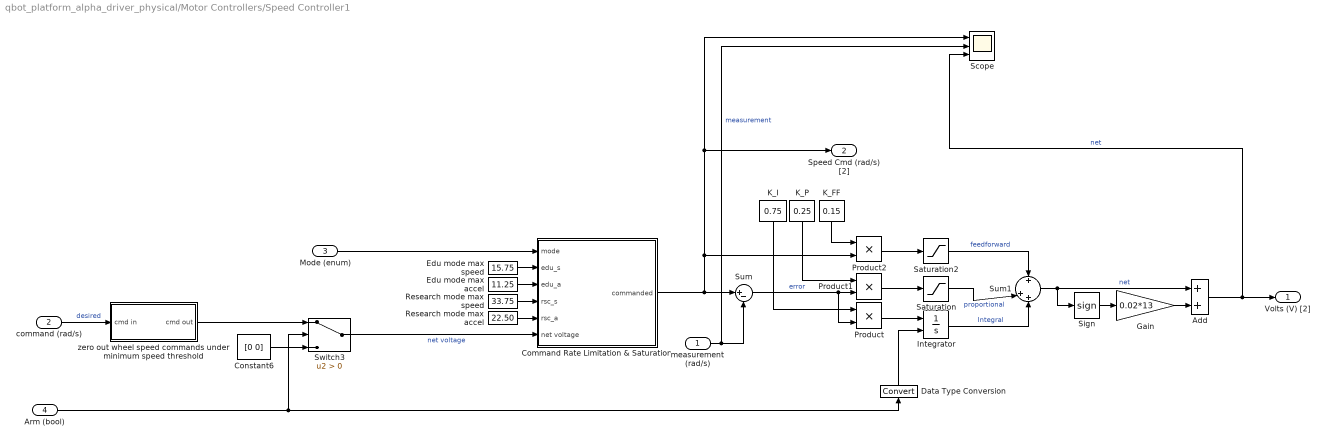
== system qbot_platform_alpha_driver_physical/Motor Controllers/Speed Controller1 ==
  measurement (rad/s) : Inport
  command (rad/s) : Inport  Port=2
  Mode (enum) : Inport  Port=3
  Arm (bool) : Inport  Port=4
  Add : Sum
  Command Rate Limitation & Saturation : Subsystem
  Constant6 : Constant  Value=[0 0]
  Data Type Conversion : DataTypeConversion  SaturateOnIntegerOverflow=off  RndMeth=Floor
  Edu mode max accel : Constant  Value=11.25
  Edu mode max speed : Constant  Value=15.75
  Gain : Gain  Gain=0.02*13
  Integrator : Integrator  ExternalReset=either  InitialCondition=[0 0]  LimitOutput=on  UpperSaturationLimit=[2 2]  LowerSaturationLimit=[-2 -2]
  K_FF : Constant  Value=0.15
  K_I : Constant  Value=0.75
  K_P : Constant  Value=0.25
  Product : Product
  Product1 : Product
  Product2 : Product
  Research mode max accel : Constant  Value=22.50
  Research mode max speed : Constant  Value=33.75
  Saturation : Saturate  UpperLimit=[5 5]  LowerLimit=[-5 -5]
  Saturation2 : Saturate  UpperLimit=[5 5]  LowerLimit=[-5 -5]
  Scope : Scope  NumInputPorts=3
  Sign : Signum
  Sum : Sum  Inputs=|+-
  Sum1 : Sum  Inputs=+|++
  Switch3 : Switch  Criteria=u2 > Threshold  SaturateOnIntegerOverflow=off  InputSameDT=off
  zero out wheel speed commands under minimum speed threshold : Subsystem
  Volts (V) [2] : Outport
  Speed Cmd (rad/s) [2] : Outport  Port=2
  wires:
  Product1/1 -> Saturation/1
  Product/1 -> Integrator/1
  Integrator/1 -> Sum1/3  "Integral"
  Sum/1 -> Product/2, Product1/2  "error"
  measurement (rad/s)/1 -> Sum/2, Scope/2  "measurement"
  command (rad/s)/1 -> zero out wheel speed commands under minimum speed threshold/1(cmd in)  "desired"
  Data Type Conversion/1 -> Integrator/2
  Add/1 -> Scope/3, Volts (V) [2]/1  "net"
  Arm (bool)/1 -> Data Type Conversion/1, Switch3/2
  Product2/1 -> Saturation2/1
  zero out wheel speed commands under minimum speed threshold/1(cmd out) -> Switch3/1
  Constant6/1 -> Switch3/3
  Command Rate Limitation & Saturation/1(commanded) -> Scope/1, Speed Cmd (rad/s) [2]/1, Product2/2, Sum/1
  Mode (enum)/1 -> Command Rate Limitation & Saturation/1(mode)
  Edu mode max speed/1 -> Command Rate Limitation & Saturation/2(edu_s)
  Edu mode max accel/1 -> Command Rate Limitation & Saturation/3(edu_a)
  Research mode max speed/1 -> Command Rate Limitation & Saturation/4(rsc_s)
  Research mode max accel/1 -> Command Rate Limitation & Saturation/5(rsc_a)
  Switch3/1 -> Command Rate Limitation & Saturation/6(net voltage)  "net voltage"
  K_I/1 -> Product/1
  K_P/1 -> Product1/1
  K_FF/1 -> Product2/1
  Saturation/1 -> Sum1/2  "proportional"
  Saturation2/1 -> Sum1/1  "feedforward"
  Sum1/1 -> Sign/1, Add/1  "net"
  Sign/1 -> Gain/1
  Gain/1 -> Add/2

== system qbot_platform_alpha_driver_physical/Motor Controllers/find hold command ==
  measurement (rad) : Inport
  Trigger : TriggerPort  VariantControl=(inherit)
  command (rad) : Outport
  wires:
  measurement (rad)/1 -> command (rad)/1

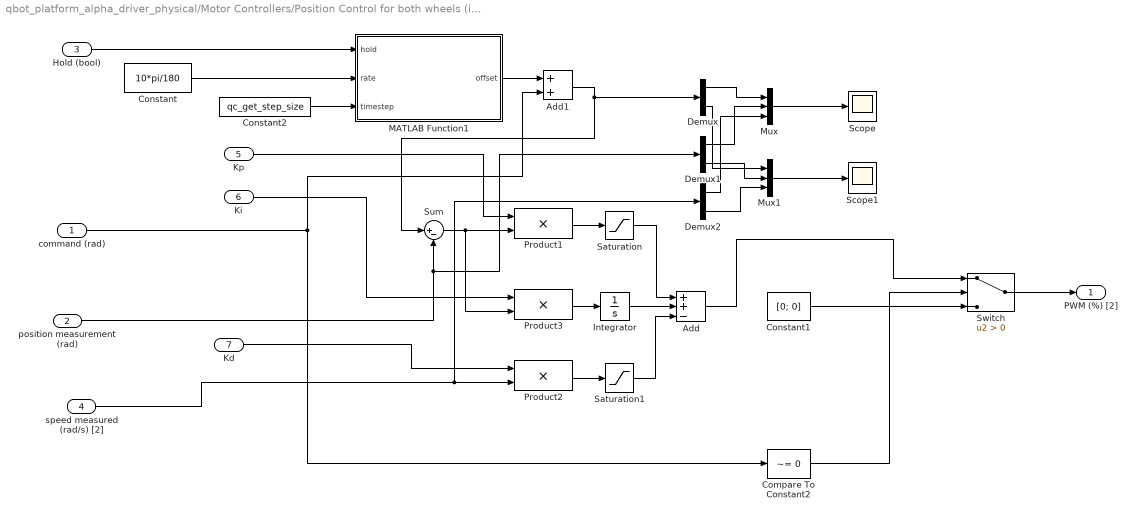
== system qbot_platform_alpha_driver_physical/Motor Controllers/Position Control for both wheels (in dev)/Drive Controller ==
  command (rad) : Inport
  position measurement (rad) : Inport  Port=2
  Hold (bool) : Inport  Port=3
  speed measured (rad/s) [2] : Inport  Port=4
  Kp : Inport  Port=5
  Ki : Inport  Port=6
  Kd : Inport  Port=7
  Add : Sum  Inputs=++-
  Add1 : Sum
  Compare To Constant2 : simulink/Logic and Bit Operations/Compare To Constant  relop=~=  const=0  OutDataTypeStr=boolean
  Constant : Constant  Value=10*pi/180
  Constant1 : Constant  Value=[0; 0]  VectorParams1D=off
  Constant2 : Constant  Value=qc_get_step_size
  Demux : Demux  Outputs=2
  Demux1 : Demux  Outputs=2
  Demux2 : Demux  Outputs=2
  Integrator : Integrator  InitialCondition=[0 0]  LimitOutput=on  UpperSaturationLimit=[0.5 0.5]  LowerSaturationLimit=[-0.5 -0.5]
  MATLAB Function1 : MATLAB Function  TreatAsAtomicUnit=on
  Mux : Mux  Inputs=3
  Mux1 : Mux  Inputs=3
  Product1 : Product
  Product2 : Product
  Product3 : Product
  Saturation : Saturate  UpperLimit=[0.7; 0.7]  LowerLimit=[-0.7; -0.7]
  Saturation1 : Saturate  UpperLimit=[0.7; 0.7]  LowerLimit=[-0.7; -0.7]
  Scope : Scope
  Scope1 : Scope
  Sum : Sum  Inputs=|+-
  Switch : Switch  Criteria=u2 > Threshold  SaturateOnIntegerOverflow=off  InputSameDT=off
  PWM (%) [2] : Outport
  wires:
  Compare To Constant2/1 -> Switch/2
  Kp/1 -> Product1/1
  Constant1/1 -> Switch/3
  Product1/1 -> Saturation/1
  Add/1 -> Switch/1
  position measurement (rad)/1 -> Demux1/1, Sum/2
  command (rad)/1 -> Compare To Constant2/1, Add1/2
  Saturation/1 -> Add/1
  Hold (bool)/1 -> MATLAB Function1/1(hold)
  Constant2/1 -> MATLAB Function1/3(timestep)
  Kd/1 -> Product2/1
  speed measured (rad/s) [2]/1 -> Demux2/1, Product2/2
  Product2/1 -> Saturation1/1
  Saturation1/1 -> Add/3
  Product3/1 -> Integrator/1
  Integrator/1 -> Add/2
  Ki/1 -> Product3/1
  Sum/1 -> Product3/2, Product1/2
  Constant/1 -> MATLAB Function1/2(rate)
  Add1/1 -> Sum/1, Demux/1
  Mux/1 -> Scope/1
  Demux/1 -> Mux/1
  Demux1/1 -> Mux/2
  Demux2/1 -> Mux/3
  Mux1/1 -> Scope1/1
  Demux1/2 -> Mux1/2
  Demux2/2 -> Mux1/3
  Demux/2 -> Mux1/1
  Switch/1 -> PWM (%) [2]/1
  MATLAB Function1/1(offset) -> Add1/1

== system qbot_platform_alpha_driver_physical/Motor Controllers/Position Control for both wheels (in dev)/find hold command1 ==
  measurement (rad) : Inport
  Trigger : TriggerPort  VariantControl=(inherit)
  command (rad) : Outport
  wires:
  measurement (rad)/1 -> command (rad)/1

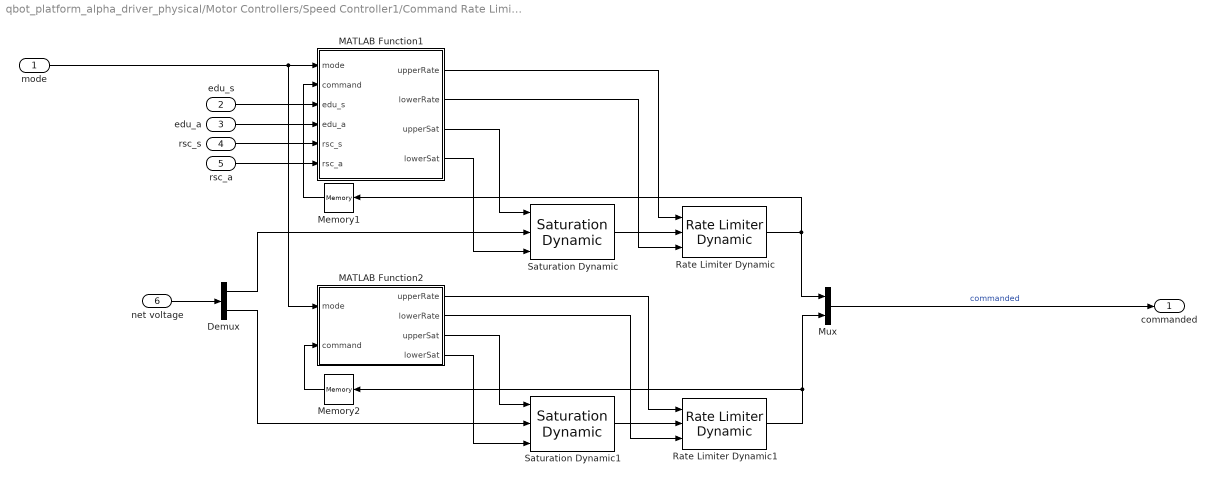
== system qbot_platform_alpha_driver_physical/Motor Controllers/Speed Controller1/Command Rate Limitation & Saturation ==
  mode : Inport
  edu_s : Inport  Port=2
  edu_a : Inport  Port=3
  rsc_s : Inport  Port=4
  rsc_a : Inport  Port=5
  net voltage : Inport  Port=6
  Demux : Demux  Outputs=2
  MATLAB Function1 : MATLAB Function  TreatAsAtomicUnit=on
  MATLAB Function2 : MATLAB Function  TreatAsAtomicUnit=on
  Memory1 : Memory
  Memory2 : Memory
  Mux : Mux  Inputs=2
  Rate Limiter Dynamic : simulink/Discontinuities/Rate Limiter Dynamic
  Rate Limiter Dynamic1 : simulink/Discontinuities/Rate Limiter Dynamic
  Saturation Dynamic : simulink/Discontinuities/Saturation Dynamic  OutMin=[]  OutMax=[]  OutDataTypeStr=Inherit: Same as second input  OutDataType=fixdt(1, 16)  OutScaling=2^-10  DoSatur=off
  Saturation Dynamic1 : simulink/Discontinuities/Saturation Dynamic  OutMin=[]  OutMax=[]  OutDataTypeStr=Inherit: Same as second input  OutDataType=fixdt(1, 16)  OutScaling=2^-10  DoSatur=off
  commanded : Outport
  wires:
  edu_s/1 -> MATLAB Function1/3(edu_s)
  MATLAB Function2/3(upperSat) -> Saturation Dynamic1/1
  Demux/2 -> Saturation Dynamic1/2
  Rate Limiter Dynamic/1 -> Memory1/1, Mux/1
  Demux/1 -> Saturation Dynamic/2
  MATLAB Function2/2(lowerRate) -> Rate Limiter Dynamic1/3
  mode/1 -> MATLAB Function2/1(mode), MATLAB Function1/1(mode)
  Rate Limiter Dynamic1/1 -> Mux/2, Memory2/1
  MATLAB Function1/3(upperSat) -> Saturation Dynamic/1
  MATLAB Function1/4(lowerSat) -> Saturation Dynamic/3
  MATLAB Function2/1(upperRate) -> Rate Limiter Dynamic1/1
  Saturation Dynamic1/1 -> Rate Limiter Dynamic1/2
  rsc_s/1 -> MATLAB Function1/5(rsc_s)
  Memory1/1 -> MATLAB Function1/2(command)
  MATLAB Function2/4(lowerSat) -> Saturation Dynamic1/3
  Saturation Dynamic/1 -> Rate Limiter Dynamic/2
  MATLAB Function1/1(upperRate) -> Rate Limiter Dynamic/1
  MATLAB Function1/2(lowerRate) -> Rate Limiter Dynamic/3
  Memory2/1 -> MATLAB Function2/2(command)
  Mux/1 -> commanded/1  "commanded"
  edu_a/1 -> MATLAB Function1/4(edu_a)
  rsc_a/1 -> MATLAB Function1/6(rsc_a)
  net voltage/1 -> Demux/1

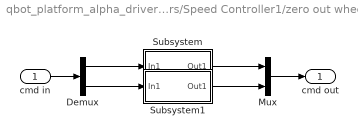
== system qbot_platform_alpha_driver_physical/Motor Controllers/Speed Controller1/zero out wheel speed commands under minimum speed threshold ==
  cmd in : Inport
  Demux : Demux  Outputs=2
  Mux : Mux  Inputs=2
  Subsystem : Subsystem
  Subsystem1 : Subsystem
  cmd out : Outport
  wires:
  cmd in/1 -> Demux/1
  Demux/1 -> Subsystem/1(In1)
  Demux/2 -> Subsystem1/1(In1)
  Subsystem/1(Out1) -> Mux/1
  Subsystem1/1(Out1) -> Mux/2
  Mux/1 -> cmd out/1

== system qbot_platform_alpha_driver_physical/Motor Controllers/Speed Controller1/zero out wheel speed commands under minimum speed threshold/Subsystem ==
  In1 : Inport
  Abs : Abs  SaturateOnIntegerOverflow=off
  Compare To Constant : simulink/Logic and Bit Operations/Compare To Constant  relop=<  const=pi/8  OutDataTypeStr=boolean
  Constant : Constant  Value=0
  Switch : Switch  Criteria=u2 > Threshold  SaturateOnIntegerOverflow=off  InputSameDT=off
  Out1 : Outport
  wires:
  In1/1 -> Switch/3, Abs/1
  Abs/1 -> Compare To Constant/1
  Compare To Constant/1 -> Switch/2
  Constant/1 -> Switch/1
  Switch/1 -> Out1/1

== system qbot_platform_alpha_driver_physical/Motor Controllers/Speed Controller1/zero out wheel speed commands under minimum speed threshold/Subsystem1 ==
  In1 : Inport
  Abs : Abs  SaturateOnIntegerOverflow=off
  Compare To Constant : simulink/Logic and Bit Operations/Compare To Constant  relop=<  const=pi/8  OutDataTypeStr=boolean
  Constant : Constant  Value=0
  Switch : Switch  Criteria=u2 > Threshold  SaturateOnIntegerOverflow=off  InputSameDT=off
  Out1 : Outport
  wires:
  Switch/1 -> Out1/1
  Constant/1 -> Switch/1
  Compare To Constant/1 -> Switch/2
  Abs/1 -> Compare To Constant/1
  In1/1 -> Abs/1, Switch/3

== matlab function qbot_platform_alpha_driver_physical/Motor Controllers/Position Control for both wheels (in dev)/Drive Controller/MATLAB Function1 ==
  data: hold input; offset output; rate input; timestep input
function offset = ramp(hold, rate, timestep)

persistent t
if isempty(t)
    t = 0;
end

if hold
    t = t + timestep;
    offset = rate * t;
else
    t = 0;
    offset = 0;
end

end

== matlab function qbot_platform_alpha_driver_physical/LED States/LEDs/MATLAB Function1 ==
  data: t input; y output; d input; p input
function y = fcn(t, d, p)

t = mod(t, p);

if t/p < d
    y = 1;
else
    y = 0;
end

== matlab function qbot_platform_alpha_driver_physical/Motor Controllers/Speed Controller1/Command Rate Limitation & Saturation/MATLAB Function1 ==
  data: mode input; command input; upperRate output; lowerRate output; upperSat output; lowerSat output; edu_s input; edu_a input; rsc_s input; rsc_a input
function [upperRate, lowerRate, upperSat, lowerSat] = fcn(mode, command, edu_s, edu_a, rsc_s, rsc_a)
% this function sets upper/lower saturation/rate limits for wheel speeds

% set acceleration and speed limits based on mode
if mode == 0 || mode == 1
    % education mode (0 and 1)
    accel_limit = edu_a; % rad/s/s
    speed_limit = edu_s; % rad/s
else
    % research mode (2 and 3)
    accel_limit = rsc_a; % rad/s/s
    speed_limit = rsc_s; % rad/s
end

% saturate the speeds the same way based on mode
upperSat    =  speed_limit;
lowerSat    = -speed_limit;

% saturate the accelerations (rate limit) based on speed commands
% to always allow faster braking
if command > 0
    upperRate =      accel_limit;
    lowerRate =  -10*accel_limit;
elseif command < 0 
    upperRate =   10*accel_limit;
    lowerRate =     -accel_limit;
else
    upperRate =      accel_limit;
    lowerRate =     -accel_limit;
end

== matlab function qbot_platform_alpha_driver_physical/LED States/LEDs/MATLAB Function2 ==
  data: t input; y output; d input; p input
function y = fcn(t, d, p)

t = mod(t, p);

if t/p < d
    y = 1;
else
    y = 0;
end

== matlab function qbot_platform_alpha_driver_physical/I//O/battery monitoring/Figure out which battery is valid and active1 ==
  data: bat_voltage output; bat_voltage_percentage output; bat input; battery_status input; low_battery output; min_bat_threshold input; max_bat_threshold input; low_bat_threshold input; stop output
function [bat_voltage, bat_voltage_percentage, low_battery, stop] = fcn(bat, battery_status, min_bat_threshold, max_bat_threshold, low_bat_threshold)

stop = 0;
low_battery = 0;
bat_voltage = 13.5;

if battery_status(1) && battery_status(2)
    bat_voltage = (bat(1) + bat(2)) / 2;
elseif battery_status(1)
    bat_voltage = bat(1);
elseif battery_status(2)
    bat_voltage = bat(2);
end

if bat_voltage <= low_bat_threshold
    low_battery = 1;
end

if bat_voltage <= min_bat_threshold
    stop = 1;
end

bat_voltage_percentage = bat_voltage / max_bat_threshold;

== matlab function qbot_platform_alpha_driver_physical/LED States/LEDs/MATLAB Function3 ==
  data: t input; y output; d input; p input
function y = fcn(t, d, p)

t = mod(t, p);

if t/p < d
    y = 1;
else
    y = 0;
end

== matlab function qbot_platform_alpha_driver_physical/From Client/MATLAB Function ==
  data: wL output; vC input; wR output; Omega input
function [wL, wR] = invKin(vC , Omega)

% wheelbase
d=0.3928; 

% calculate wheel linear velocities
vR = vC + Omega*d/2;
vL = vC - Omega*d/2;

% calculate wheel angular velocities
wheelRadius = 3.5*0.0254/2;

wR = vR/ wheelRadius;
wL = vL/ wheelRadius;

== matlab function qbot_platform_alpha_driver_physical/I//O/battery monitoring/Figure out which battery is valid and active ==
  data: bat input; low_battery output; active output; min_bat_threshold input; max_bat_threshold input; low_bat_threshold input
function [low_battery, active] = fcn(bat, min_bat_threshold, max_bat_threshold, low_bat_threshold)
low_battery = [0, 0];
valid = [bat(1) > min_bat_threshold && bat(1) < max_bat_threshold , bat(2) > min_bat_threshold && bat(2) < max_bat_threshold];

if valid(1) && valid(2)
    if bat(1) < bat(2)
        active = 1;
    else
        active = 2;
    end
elseif valid(1)
    active = 1;
elseif valid(2)
    active = 2;
else
    active = 0;
end

if bat(1) < low_bat_threshold && valid(1)
    low_battery(1) = 1;
end

if bat(2) < low_bat_threshold && valid(2)
    low_battery(2) = 1;
end

== matlab function qbot_platform_alpha_driver_physical/Motor Controllers/Speed Controller1/Command Rate Limitation & Saturation/MATLAB Function2 ==
  data: mode input; command input; upperRate output; lowerRate output; upperSat output; lowerSat output
function [upperRate, lowerRate, upperSat, lowerSat] = fcn(mode, command)
% this function sets upper/lower saturation/rate limits for wheel speeds

% set acceleration and speed limits based on mode
if mode == 0 || mode == 1
    % education mode (0 and 1)
    accel_limit = 11.25; % rad/s/s
    speed_limit = 15.75; % rad/s
else
    % research mode (2 and 3)
    accel_limit = 22.50; % rad/s/s
    speed_limit = 33.75; % rad/s
end

% saturate the speeds the same way based on mode
upperSat    =  speed_limit;
lowerSat    = -speed_limit;

% saturate the accelerations (rate limit) based on speed commands
% to always allow faster braking
if command > 0
    upperRate =      accel_limit;
    lowerRate =  -10*accel_limit;
elseif command < 0 
    upperRate =   10*accel_limit;
    lowerRate =     -accel_limit;
else
    upperRate =      accel_limit;
    lowerRate =     -accel_limit;
end
